simulink model "Pitch_Actuation_Hydraulic_Testrig_rt"  (Simulink 7.9)
settings: Solver=ode15s  StartTime=0.0  StopTime=10.0  RelTol=1e-3
PostLoadFcn:
  | warning off xPCTarget:sampleTime:sampleTimeInvariance;
  | warning off Simulink:SL_MdlFileShadowedByFile;
StartFcn:
  | tic;
StopFcn:
  | Elapsed_Sim_Time = toc; disp(['Elapsed time is ' num2str(Elapsed_Sim_Time)])
undefined symbols (not defined in the file or in its folder): sigbuilder_block, WT_Params
libraries: fl_lib x20, mblibv1 x12, nesl_utility x10, sh_lib x9, xpclib x1
Description:
  | Copyright 2011 The MathWorks, Inc.
settings Model: Creator=smiller  LastModifiedBy=smiller  ExtModeTrigDuration=200  BufferReuse=off
settings SolverCC: ExtrapolationOrder=2  NumberNewtonIterations=2  MaxConsecutiveMinStep=3
settings DataIOCC: LimitDataPoints=off
settings OptimizationCC: BlockReduction=off  OptimizeBlockIOStorage=off  BufferReuse=off  ExpressionFolding=off  LocalBlockOutputs=off
settings DebuggingCC: SolverPrmCheckMsg=none  FcnCallInpInsideContextMsg=Use local settings  UnconnectedInputMsg=none  UnconnectedOutputMsg=none  StrictBusMsg=Warning
settings HardwareCC: ProdIntDivRoundTo=Zero  ProdEndianess=LittleEndian  ProdHWDeviceType=Generic->32-bit x86 compatible
settings RTWCC: SystemTargetFile=xpctarget.tlc  TemplateMakefile=xpc_default_tmf  Description=xPC Target  ProcessScript=xpctarget_make_rtw_hook  RTWCompilerOptimization=On
settings xpcTargetCC: TargetFcnLib=ansi_tfl_table_tmw.mat  CodeReplacementLibrary=XPC_BLAS  CodeExecutionProfiling=off  ParMdlRefBuildCompliant=on  ConcurrentExecutionCompliant=on  CombineSignalStateStructs=off  PortableWordSizes=off  GRTInterface=on  xPCTaskExecutionProfile=off  xPCRL32EventNumber=5000  xPCLoadParamSetFile=off  xPCConcurrentTasks=off  xPCEnableSFAnimation=off
settings SimscapeCC: ExplicitSolverDiagnosticOptions=none
settings SimMechanicsCC: WarnOnRedundantConstraints=off  VisSampleTime=0.1  AnimationDelay=0  LastVizWinPosition=[420 528 560 420]  CamPosition=[-0.6;-13.224;-0.5;]  CamTarget=[-0.6;19.95;-0.5;]  CamUpVector=[0;0;1;]  CamHeight=3.468  VisBackgroundColor=[0.9;0.9;0.95;]  DefaultBodyColor=[1;0;0;]
settings ConfigurationSet: Description=SimMechanics 2G

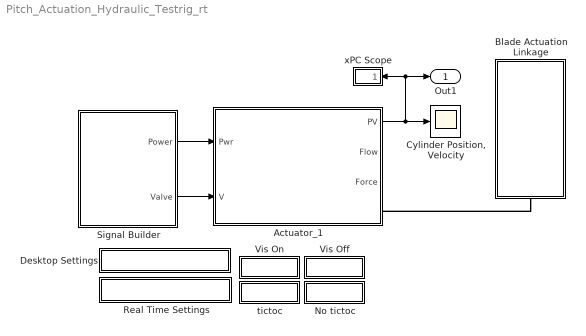
== system Pitch_Actuation_Hydraulic_Testrig_rt ==
  Actuator_1 : Subsystem
      mask Display: image(imread('Pitch_Hydraulic_Actuator_IMAGE.jpg'));
  Blade Actuation Linkage : Subsystem
      mask Display: image(imread('Single_Blade_IMAGE.jpg'));
  "Cylinder Position, Velocity" : Scope
      settings: TimeRange=10  YMin=-0.4  YMax=0.6  SaveName=Hydraulic_Testrig_DATA
  Desktop Settings : Subsystem
      settings: OpenFcn=|
      | set_param(bdroot,'Solver','ODE15s','MaxStep','auto');
      | 
      | tvar_solverBlock = find_system(bdroot, 'SubClassName', 'solver');
      | 
      | for i=1:size(tvar_solverBlock,1)
      | 
      | set_param(char(tvar_solverBlock(i)), 'UseLocalSolver','off','DoFixedCost','off');
      | end
      | 
      | clear tvar_solverBlock
      mask Display: disp('Desktop Settings')
  No tictoc : Subsystem
      settings: OpenFcn=|
      | set_param(bdroot,'StartFcn','');
      | set_param(bdroot,'StopFcn','');
      mask Display: disp('No tictoc')
  Real Time Settings : Subsystem
      settings: OpenFcn=|
      | tvar_Nonlinear_Iterations = '3';
      | 
      | tvar_StepSize = '0.005';
      | 
      | %tvar_LocalSolver = 'NE_TRAPEZOIDAL_ADVANCER';
      | 
      | tvar_LocalSolver = 'NE_BACKWARD_EULER_ADVANCER';
      | 
      | set_param(bdroot,'Solver','ode3','FixedStep','auto');
      | 
      | tvar_solverBlock = find_system(bdroot, 'SubClassName', 'solver');
      | for i=1:size(tvar_solverBlock,1)
      | 
      | set_param(char(tvar_solverBlock(i)), 'UseLocalSolver','on','DoFixedCost','on','MaxNonlinIter',tvar_Nonlinear_Iterations,'LocalSolverChoice',tvar_LocalSolver,'LocalSolverSampleTime',tvar_StepSize);
      | end
      | clear tvar_Nonlinear_Iterations tvar_StepSize tvar_LocalSolver tvar_solverBlock
      mask Display: disp('Real Time Settings')
  Signal Builder : Subsystem  Tag=STV Subsys  LoadFcn=sigbuilder_block('load');  StartFcn=sigbuilder_block('start');  StopFcn=sigbuilder_block('stop');  ClipboardFcn=sigbuilder_block('clipboard');  mask(Sigbuilder block){}
      mask help: Sigbuilder GUI
      mask init:
      | if ~strcmp(get_param(bdroot(gcbh),'SimulationStatus'),'stopped') tuvar = sigbuilder_block('maskInit'); end
      settings: CopyFcn=sigbuilder_block('copy');  DeleteFcn=sigbuilder_block('delete');  ModelCloseFcn=sigbuilder_block('modelClose');  PreSaveFcn=sigbuilder_block('preSave');  PauseFcn=sigbuilder_block('pause')  ContinueFcn=sigbuilder_block('continue')  NameChangeFcn=sigbuilder_block('namechange');  OpenFcn=sigbuilder_block('open',[141.75 274.5 550.5 399.75 ]);  CloseFcn=sigbuilder_block('close');
      mask Display: plot(0,0,100,100,[10,10,40,40,10],[80,20,20,80,80],[40,10],[50,50], [40,27,10],[65,72,56],[40,25,25,10],[28,28,43,43]);
  Vis Off : Subsystem
      settings: OpenFcn=|
      | Temp_ENVHa= get_param(find_system(gcs,'LookUnderMasks','all','FollowLinks','on','ClassName','Environment'),'handle');
      | 
      | set_param(Temp_ENVHa{1},'VisualizeMachine','off');
      | 
      | set_param(gcs,'VisDuringSimulation','off')
      | set_param(gcs,'VisOnUpdateDiagram','off')
      mask Display: disp('Vis Off')
  Vis On : Subsystem
      settings: OpenFcn=|
      | Temp_ENVHa= get_param(find_system(gcs,'LookUnderMasks','all','FollowLinks','on','ClassName','Environment'),'handle');
      | 
      | set_param(Temp_ENVHa{1},'VisualizeMachine','on');
      | clear Temp_ENVHa;
      | set_param(gcs,'VisDuringSimulation','on')
      | set_param(gcs,'VisOnUpdateDiagram','on')
      mask Display: disp('Vis On')
  tictoc : Subsystem
      settings: OpenFcn=|
      | set_param(bdroot,'StartFcn','tic;');
      | set_param(bdroot,'StopFcn','Elapsed_Sim_Time = toc; disp([''Elapsed time is '' num2str(Elapsed_Sim_Time)])');
      mask Display: disp('tictoc')
  xPC Scope : Subsystem
      mask Display: disp('xPC')
  Out1 : Outport
  wires:
  Signal Builder/1(Power) -> Actuator_1/1(Pwr)
  Signal Builder/2(Valve) -> Actuator_1/2(V)
  Actuator_1/1(PV) -> "Cylinder Position, Velocity"/1, Out1/1, xPC Scope/1(In1)
  connections:
  Blade Actuation Linkage/LConn1 -- Actuator_1/RConn1

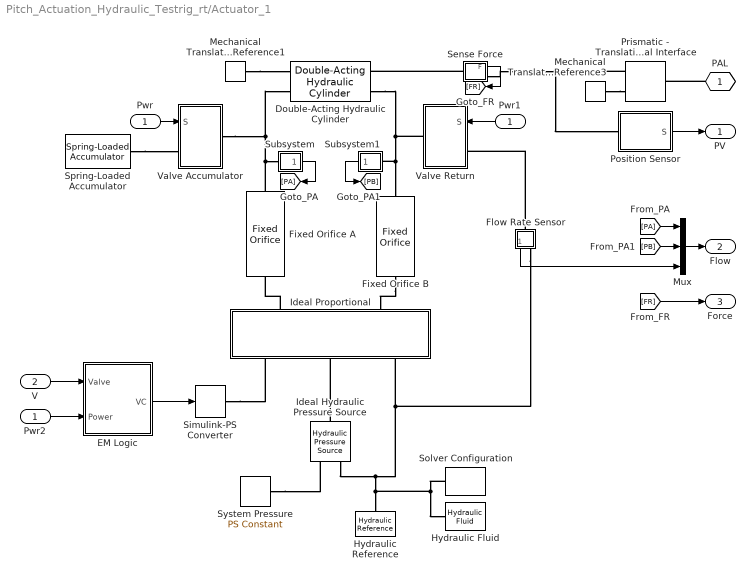
== system Pitch_Actuation_Hydraulic_Testrig_rt/Actuator_1 ==
  Pwr : Inport
  V : Inport  Port=2
  Double-Acting Hydraulic Cylinder : sh_lib/Hydraulic Cylinders/Double-Acting Hydraulic Cylinder  area_A=WT_Params.Pitch_Actuator.Cylinder.piston_area m^2  area_B=WT_Params.Pitch_Actuator.Cylinder.piston_area m^2  stroke=WT_Params.Pitch_Actuator.Cylinder.stroke m  init_pos=WT_Params.Pitch_Actuator.Cylinder.initial_disp_from_a m  dead_vol_A=1e-04 m^3  dead_vol_B=1e-04 m^3  init_pressure_A=0 Pa  init_pressure_B=0 Pa  k_sh=1.4  stiff=WT_Params.Pitch_Actuator.Cylinder.contact_stiffness N/m  D=WT_Params.Pitch_Actuator.Cylinder.contact_damping N/(m/s)  or=2  LocalVarLogging=[]
  EM Logic : Subsystem
  Fixed Orifice A : sh_lib/Orifices/Fixed Orifice  area=WT_Params.Pitch_Actuator.orifice_area m^2  C_d=0.7  Re_cr=12  flow_rate_Log=off  pr_drop_Log=off  Re_Log=off  power_Log=off  LocalVarNames=|flow_rate|pr_drop|Re|power  LocalVarDescs=|Flow rate through the orifice (m^3/s)|Pressure drop across the orifice (Pa)|Reynolds number|Power (W)  LocalVarLogging=[0 0 0 0]
  Fixed Orifice B : sh_lib/Orifices/Fixed Orifice  area=WT_Params.Pitch_Actuator.orifice_area m^2  C_d=0.7  Re_cr=12  flow_rate_Log=off  pr_drop_Log=off  Re_Log=off  power_Log=off  LocalVarNames=|flow_rate|pr_drop|Re|power  LocalVarDescs=|Flow rate through the orifice (m^3/s)|Pressure drop across the orifice (Pa)|Reynolds number|Power (W)  LocalVarLogging=[0 0 0 0]
  Flow Rate Sensor : Subsystem
      mask Display: disp('F')
  Hydraulic Reference : fl_lib/Hydraulic/Hydraulic Elements/Hydraulic Reference  q_Log=off  LocalVarNames=|q  LocalVarDescs=|q  LocalVarLogging=[]
  Hydraulic Fluid : sh_lib/Hydraulic Utilities/Hydraulic Fluid  DataSource=1  SelFluid=1  SysTemp=60 c  TrapAir=0.005  ViscDerFactor=1  LocalVarLogging=[]
  Ideal Proportional : Subsystem
      mask Display:
      | plot([198.418507352471;198.418507352471], [5.66910021007061;25.5109509453177])
      | plot([189.914857037365;206.922157667577], [25.5109509453177;25.5109509453177])
      | plot([240.936758928001;240.936758928001], [5.66910021007061;25.5109509453177])
      | plot([232.433108612895;249.440409243107], [25.5109509453177;25.5109509453177])
      | plot([240.936758928001;240.936758928001], [76.5328528359532;56.6910021007061])
      | plot([232.433108612895;249.440409243107], [56.6910021007061;56.6910021007061])
      | plot([198.418507352471;198.418507352471], [76.5328528359532;56.6910021007061])
      | plot([189.914857037365;206.922157667577], [56.6910021007061;56.6910021007061])
      | plot([99.2092536762357;99.2092536762357], [76.5328528359532;5.66910021007061])
      | plot([141.727505251765;141.727505251765], [76.5328528359532;5.66910021007061])
      | plot([170.073006302118;170.073006302118], [76.5328528359532;5.66910021007061])
      | plot([269.282259978354;269.282259978354], [76.5328528359532;5.66910021007061])
      | patch([99.2092536762357;93.5401534661651;104.878353886306;99.2092536762357], [76.5328528359532;53.8564519956708;53.8564519956708;76.5328528359532],[0 0 0])
      | plot([99.2092536762357;93.5401534661651;104.878353886306;99.2092536762357], [76.5328528359532;53.8564519956708;53.8564519956708;76.5328528359532])
      | patch([141.727505251765;136.058405041695;147.396605461836;141.727505251765], [5.66910021007061;28.3455010503531;28.3455010503531;5.66910021007061],[0 0 0])
      | plot([141.727505251765;136.058405041695;147.396605461836;141.727505251765], [5.66910021007061;28.3455010503531;28.3455010503531;5.66910021007061])
      | plot([297.627761028707;340.146012604237], [5.66910021007061;76.5328528359532])
      | plot([297.627761028707;340.146012604237], [76.5328528359532;5.66910021007061])
      | plot([70.8637526258826;368.49151365459;368.49151365459;70.8637526258826;70.8637526258826], [76.5328528359532;76.5328528359532;5.66910021007061;5.66910021007061;76.5328528359532])
      | patch([297.627761028707;303.296861238778;311.800511553884;297.627761028707], [5.66910021007061;25.5109509453177;19.8418507352471;5.66910021007061],[0 0 0])
      | plot([297.627761028707;303.296861238778;311.800511553884;297.627761028707], [5.66910021007061;25.5109509453177;19.8418507352471;5.66910021007061])
      | patch([297.627761028707;303.296861238778;311.800511553884;297.627761028707], [76.5328528359532;56.6910021007061;62.3601023107767;76.5328528359532],[0 0 0])
      | plot([297.627761028707;303.296861238778;311.800511553884;297.627761028707], [76.5328528359532;56.6910021007061;62.3601023107767;76.5328528359532])
      | plot([62.3601023107767;374.16061386466], [82.2019530460238;82.2019530460238])
      | plot([65.194652415812;376.995163969696], [0;0])
      | plot([70.8637526258826;0;0;70.8637526258826;70.8637526258826], [53.8564519956708;53.8564519956708;25.5109509453177;25.5109509453177;53.8564519956708]-25.5109509453177+5.66910021007061)
      | plot([70.8637526258826;0;0;70.8637526258826;70.8637526258826]+368.49151365459, [53.8564519956708;53.8564519956708;25.5109509453177;25.5109509453177;53.8564519956708]-25.5109509453177+5.66910021007061)
      | plot([15 25], [5.66910021007061 35])
      | plot([25 15]+405, [5.66910021007061 35])
      | plot([42.5 40]+5,[70 58]);
      | plot([45 50]+2.5,[70 45]);
      | plot([45 50]+7.5,[45 70]);
      | plot([45 50]+12.5,[70 45]);
      | plot([45 50]+17.5,[45 70]);
      | plot([40 42.5]+27.5,[70 58]);
      | plot([42.5 40]+5+324,[70 58]);
      | plot([45 50]+2.5+324,[70 45]);
      | plot([45 50]+7.5+324,[45 70]);
      | plot([45 50]+12.5+324,[70 45]);
      | plot([45 50]+17.5+324,[45 70]);
      | plot([40 42.5]+27.5+324,[70 58]);
      | ;color('red');
      | port_label('LConn', 1,'A')
      | port_label('LConn', 2,'B')
      | port_label('RConn', 1,'S')
      | port_label('RConn', 2,'P')
      | port_label('RConn', 3,'T')
  Ideal Hydraulic Pressure Source : fl_lib/Hydraulic/Hydraulic Sources/Hydraulic Pressure Source  q_Log=off  p_Log=off  LocalVarNames=|flow_rate|pr_differential|power  LocalVarDescs=|Flow rate through the source (m^3/s)|Pressure differential across the source (Pa)|Source power (W)  LocalVarLogging=[0 0 0]
  Mechanical Translational Reference1 : fl_lib/Mechanical/Translational Elements/Mechanical Translational Reference  Tag=Factory Generic  f_Log=off  LocalVarNames=|f  LocalVarDescs=|f  LocalVarLogging=[]
  Mechanical Translational Reference3 : fl_lib/Mechanical/Translational Elements/Mechanical Translational Reference  Tag=Factory Generic  f_Log=off  LocalVarNames=|f  LocalVarDescs=|f  LocalVarLogging=[]
  Mux : Mux  Inputs=3
  Position Sensor : Subsystem
      mask Display:
      | plot([25.5109509453177;56.6910021007061;70.8637526258826;96.3747035712004;127.554754726589;155.900255776942;184.245756827295;212.591257877648;235.26765871793;252.274959348142;283.455010503531], [155.900255776942;155.900255776942;110.547454096377;198.418507352471;113.382004201412;198.418507352471;116.216554306448;198.418507352471;113.382004201412;155.900255776942;155.900255776942])
      | plot([155.900255776942;155.900255776942], [266.447709873319;198.418507352471])
      | patch([155.900255776942;170.073006302118;141.727505251765;155.900255776942], [198.418507352471;226.764008402824;226.764008402824;198.418507352471], [0;0;0])
      | plot([155.900255776942;170.073006302118;141.727505251765;155.900255776942], [198.418507352471;226.764008402824;226.764008402824;198.418507352471])
      | ;
      | color('red');
      | port_label('LConn', 1,'R')
      | port_label('output', 1,'P')
  Prismatic - Translational Interface : mblibv1/Interface  Elements/Prismatic - Translational Interface  UpdateFromCAD=off  DialogClass=PrismaticTranslationalInterface  Primitive=P1
  Pwr1 : InportShadow  Port=1
  Pwr2 : InportShadow  Port=1
  Sense Force : Subsystem
      mask Display: disp('F');
  Simulink-PS Converter : nesl_utility/Simulink-PS Converter  PhysicalDomain=network_engine_domain  LeftPortType=input  RightPortType=output  SubClassName=ps_input  Unit=1  AffineConversion=off  InputFilterTimeConstant=.001  UdotUserProvided=0  SimscapeFilterOrder=1  InputFiltering=off
  Solver Configuration : nesl_utility/Solver Configuration  PhysicalDomain=network_engine_domain  LeftPortType=input  RightPortType=generic  SubClassName=solver  UseCustomDae=off  DoDC=off  ResidualTolerance=WT_Params.Pitch_Actuator.constraint_tol  UseLocalSolver=off  LocalSolverChoice=NE_BACKWARD_EULER_ADVANCER  LocalSolverSampleTime=0.005  DoFixedCost=off  MaxNonlinIter=3  MaxModeIter=2  LinearAlgebra=Full  Accelerate=off  Profile=off  UseLocalSampling=off  DelaysMemoryBudget=1024
  Spring-Loaded Accumulator : sh_lib/Accumulators/Spring-Loaded Accumulator  capacity=WT_Params.Pitch_Actuator.Accumulator.capacity m^3  pr_preload=WT_Params.Pitch_Actuator.Accumulator.preload_pressure Pa  pr_max=WT_Params.Pitch_Actuator.Accumulator.maximum_pressure Pa  v_init=WT_Params.Pitch_Actuator.Accumulator.initial_volume m^3  str_compl=4e-15 m^3/Pa  flow_rate_Log=off  pr_fluid_Log=off  fluid_volume_Log=off  LocalVarNames=|flow_rate|pr_fluid|fluid_volume  LocalVarDescs=|Accumulator flow rate (m^3/s)|Fluid pressure (Pa)|Initial fluid volume (m^3)  LocalVarLogging=[0 0 0]
  Subsystem : Subsystem
      mask Display: disp('P')
  Subsystem1 : Subsystem
      mask Display: disp('P')
  System Pressure : fl_lib/Physical Signals/Sources/PS Constant  constant=WT_Params.Pitch_Actuator.hydraulic_pressure  LocalVarLogging=[]
  Valve Accumulator : Subsystem
      mask Display:
      | plot([73.6983027309179;124.720204621553], [181.41120672226;181.41120672226])
      | plot([76.2808928266168;277.78591029346], [385.498814284801;385.498814284801])
      | plot([77.0997628569603;276.967040263116], [283.455010503531;283.455010503531])
      | plot([73.6983027309179;276.967040263116;276.967040263116;73.6983027309179;73.6983027309179], [487.542618066072;487.542618066072;79.3674029409885;79.3674029409885;487.542618066072])
      | plot([277.78591029346;226.764008402824], [181.41120672226;181.285226717591])
      | plot([226.764008402824;226.764008402824], [205.28441760689;157.286035828292])
      | patch([206.35524764657;206.35524764657;280.368500389159;206.35524764657], [400.805384851992;370.192243717611;385.498814284801;400.805384851992], [0;0;0])
      | plot([206.35524764657;206.35524764657;280.368500389159;206.35524764657], [400.805384851992;370.192243717611;385.498814284801;400.805384851992])
      | plot([124.720204621553;124.720204621553], [204.906477592885;156.971085816622])
      | plot([0;351.484213024378;351.484213024378;0;0], [566.910021007061;566.910021007061;0;0;566.910021007061])
      | ;
      | color('red');
      | port_label('input', 1,'S');
      | port_label('lconn', 1,'A');
      | port_label('rconn', 1,'B');
  Valve Return : Subsystem
      mask Display:
      | plot([73.6983027309179;124.720204621553], [181.41120672226;181.41120672226])
      | plot([76.2808928266168;277.78591029346], [385.498814284801;385.498814284801])
      | plot([77.0997628569603;276.967040263116], [283.455010503531;283.455010503531])
      | plot([73.6983027309179;276.967040263116;276.967040263116;73.6983027309179;73.6983027309179], [487.542618066072;487.542618066072;79.3674029409885;79.3674029409885;487.542618066072])
      | plot([277.78591029346;226.764008402824], [181.41120672226;181.285226717591])
      | plot([226.764008402824;226.764008402824], [205.28441760689;157.286035828292])
      | patch([206.35524764657;206.35524764657;280.368500389159;206.35524764657], [400.805384851992;370.192243717611;385.498814284801;400.805384851992], [0;0;0])
      | plot([206.35524764657;206.35524764657;280.368500389159;206.35524764657], [400.805384851992;370.192243717611;385.498814284801;400.805384851992])
      | plot([124.720204621553;124.720204621553], [204.906477592885;156.971085816622])
      | plot([0;351.484213024378;351.484213024378;0;0], [566.910021007061;566.910021007061;0;0;566.910021007061])
      | ;
      | color('red');
      | port_label('input', 1,'S');
      | port_label('lconn', 1,'A');
      | port_label('rconn', 1,'B');
  PAL : PMIOPort  Tag=PMCPort  Port=1  Side=Right
  PV : Outport
  Flow : Outport  Port=2
  Force : Outport  Port=3
  wires:
  [FR] -> Force/1
  Sense Force/1(F) -> [FR]
  Mux/1 -> Flow/1
  Position Sensor/1(S) -> PV/1
  Pwr/1 -> Valve Accumulator/1(S)
  Pwr1/1 -> Valve Return/1(S)
  V/1 -> EM Logic/1(Valve)
  Subsystem/1(P) -> [PA]
  Subsystem1/1(P) -> [PB]
  Flow Rate Sensor/1(Flow) -> Mux/3
  [PA] -> Mux/1
  [PB] -> Mux/2
  EM Logic/1(VC) -> Simulink-PS Converter/1
  Pwr2/1 -> EM Logic/2(Power)
  connections:
  Sense Force/LConn1 -- Double-Acting Hydraulic Cylinder/RConn1
  PAL/RConn1 -- Prismatic - Translational Interface/RConn1
  Mechanical Translational Reference3/LConn1 -- Prismatic - Translational Interface/LConn2
  System Pressure/RConn1 -- Ideal Hydraulic Pressure Source/RConn1
  Ideal Hydraulic Pressure Source/LConn1 -- Ideal Proportional/RConn2
  Simulink-PS Converter/RConn1 -- Ideal Proportional/RConn1
  Ideal Hydraulic Pressure Source/RConn2 -- Solver Configuration/RConn1 -- Hydraulic Fluid/RConn1 -- Hydraulic Reference/LConn1 -- Flow Rate Sensor/RConn1 -- Ideal Proportional/RConn3
  Fixed Orifice B/LConn1 -- Ideal Proportional/LConn2
  Ideal Proportional/LConn1 -- Fixed Orifice A/LConn1
  Double-Acting Hydraulic Cylinder/RConn2 -- Valve Return/RConn1 -- Fixed Orifice B/RConn1 -- Subsystem1/LConn1
  Fixed Orifice A/RConn1 -- Double-Acting Hydraulic Cylinder/LConn2 -- Valve Accumulator/RConn1 -- Subsystem/LConn1
  Mechanical Translational Reference1/LConn1 -- Double-Acting Hydraulic Cylinder/LConn1
  Spring-Loaded Accumulator/RConn1 -- Valve Accumulator/LConn1
  Sense Force/RConn1 -- Position Sensor/LConn1 -- Prismatic - Translational Interface/LConn1
  Flow Rate Sensor/LConn1 -- Valve Return/LConn1

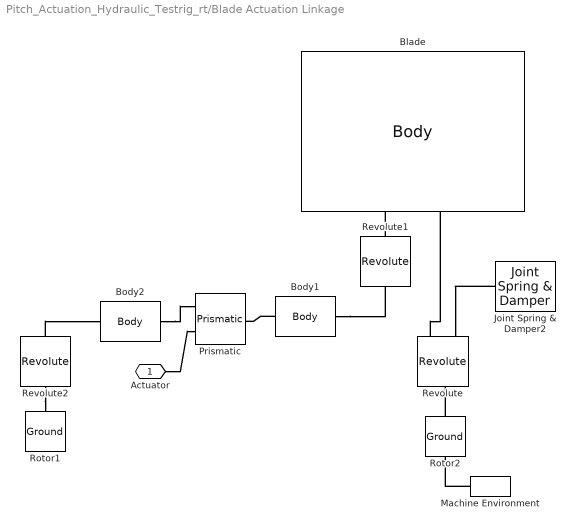
== system Pitch_Actuation_Hydraulic_Testrig_rt/Blade Actuation Linkage ==
  Blade : mblibv1/Bodies/Body  LConnTagsString=CS4|CS6|CS1|CS5  RConnTagsString=CS2  UpdateFromCAD=off  DialogClass=MechanicalBodyBlock  Mass=WT_Params.Blade.mass  MassUnits=kg  InertiaUnits=kg*m^2  Inertia=WT_Params.Blade.inertia  Shape=Cylinder  ShapeDims=[1 1]  ShapeUnits=m  ShapeUse=false  Density=1  DensityUnits=kg/m^3  DensityUse=false  GraphicsMode=MACHINE_DEFAULT  BodyColorSelMode=COLORPALETTE  BodyColor=[1 1 1]  AttachedToCS=CG  CG=Left$CG$[0 WT_Params.Blade.length/2 0]$CS1$CS1$m$[0 0 0]$Euler X-Y-Z$deg$CS1$false$none  WorkingFrames=Left$CS4$[0 0 0]$CS1$CS1$m$[0 0 0]$Euler X-Y-Z$deg$CS1$true$none#Left$CS6$[WT_Params.Blade.Actuator_Offset.x WT_Params.Blade.Actuator_Offset.y WT_Params.Blade.Actuator_Offset.z]$CS1$CS1$m$[0 0 0]$Euler X-Y-Z$deg$CS1$true$none#Left$CS1$[0 0 0]$Adjoining$Adjoining$m$[0 0 0]$Euler X-Y-Z$deg$Adjoining$true$none#Left$CS7$[WT_Params.Blade.Geometry.root_radius*sin(0) 0 WT_Params.Blade.Geometry.root_radius*cos(0)]$CS1$CS1$m$[0 0 0]$Euler X-Y-Z$deg$CS1$false$none#Left$CS8$[WT_Params.Blade.Geometry.root_radius*sin(0.2*pi) 0 WT_Params.Blade.Geometry.root_radius*cos(0.2*pi)]$CS1$CS1$m$[0 0 0]$Euler X-Y-Z$deg$CS1$false$none#Left$CS9$[WT_Params.Blade.Geometry.root_radius*sin(0.4*pi) 0 WT_Params.Blade.Geometry.root_radius*cos(0.4*pi)]$CS1$CS1$m$[0 0 0]$Euler X-Y-Z$deg$CS1$false$none#Left$CS10$[WT_Params.Blade.Geometry.root_radius*sin(0.6*pi) 0 WT_Params.Blade.Geometry.root_radius*cos(0.6*pi)]$CS1$CS1$m$[0 0 0]$Euler X-Y-Z$deg$CS1$false$none#Left$CS11$[WT_Params.Blade.Geometry.root_radius*sin(0.8*pi) 0 WT_Params.Blade.Geometry.root_radius*cos(0.8*pi)]$CS1$CS1$m$[0 0 0]$Euler X-Y-Z$deg$CS1$false$none#Left$CS12$[WT_Params.Blade.Geometry.root_radius*sin(1.0*pi) 0 WT_Params.Blade.Geometry.root_radius*cos(1.0*pi)]$CS1$CS1$m$[0 0 0]$Euler X-Y-Z$deg$CS1$false$none#Left$CS13$[WT_Params.Blade.Geometry.root_radius*sin(1.2*pi) 0 WT_Params.Blade.Geometry.root_radius*cos(1.2*pi)]$CS1$CS1$m$[0 0 0]$Euler X-Y-Z$deg$CS1$false$none#Left$CS14$[WT_Params.Blade.Geometry.root_radius*sin(1.4*pi) 0 WT_Params.Blade.Geometry.root_radius*cos(1.4*pi)]$CS1$CS1$m$[0 0 0]$Euler X-Y-Z$deg$CS1$false$none#Left$CS15$[WT_Params.Blade.Geometry.root_radius*sin(1.6*pi) 0 WT_Params.Blade.Geometry.root_radius*cos(1.6*pi)]$CS1$CS1$m$[0 0 0]$Euler X-Y-Z$deg$CS1$false$none#Left$CS16$[WT_Params.Blade.Geometry.root_radius*sin(1.8*pi) 0 WT_Params.Blade.Geometry.root_radius*cos(1.8*pi)]$CS1$CS1$m$[0 0 0]$Euler X-Y-Z$deg$CS1$false$none#Left$CS17$[0 WT_Params.Blade.length/4 0]$CS1$CS1$m$[0 0 0]$Euler X-Y-Z$deg$CS1$false$none#Left$CS18$[WT_Params.Blade.Geometry.ctr_to_leading_edge.x 0 WT_Params.Blade.Geometry.ctr_to_leading_edge.z]$CS17$CS17$m$[0 0 0]$Euler X-Y-Z$deg$CS1$false$none#Left$CS19$[WT_Params.Blade.Geometry.ctr_to_a1.x 0 WT_Params.Blade.Geometry.ctr_to_a1.z]$CS17$CS17$m$[0 0 0]$Euler X-Y-Z$deg$CS1$false$none#Left$CS20$[WT_Params.Blade.Geometry.ctr_to_a2.x 0 WT_Params.Blade.Geometry.ctr_to_a2.z]$CS17$CS17$m$[0 0 0]$Euler X-Y-Z$deg$CS1$false$none#Left$CS21$[WT_Params.Blade.Geometry.ctr_to_b1.x 0 WT_Params.Blade.Geometry.ctr_to_b1.z]$CS17$CS17$m$[0 0 0]$Euler X-Y-Z$deg$CS1$false$none#Left$CS25$[WT_Params.Blade.Geometry.ctr_to_b2.x 0 WT_Params.Blade.Geometry.ctr_to_b2.z]$CS17$CS17$m$[0 0 0]$Euler X-Y-Z$deg$CS1$false$none#Left$CS22$[WT_Params.Blade.Geometry.ctr_to_c1.x 0 WT_Params.Blade.Geometry.ctr_to_c1.z]$CS17$CS17$m$[0 0 0]$Euler X-Y-Z$deg$CS1$false$none#Left$CS3$[WT_Params.Blade.Geometry.ctr_to_d1.x 0 WT_Params.Blade.Geometry.ctr_to_d1.z]$CS17$CS17$m$[0 0 0]$Euler X-Y-Z$deg$CS1$false$none#Left$CS23$[WT_Params.Blade.Geometry.ctr_to_e1.x 0 WT_Params.Blade.Geometry.ctr_to_e1.z]$CS17$CS17$m$[0 0 0]$Euler X-Y-Z$deg$CS1$false$none#Left$CS24$[WT_Params.Blade.Geometry.ctr_to_trailing_edge.x 0 WT_Params.Blade.Geometry.ctr_to_trailing_edge.z]$CS17$CS17$m$[0 0 0]$Euler X-Y-Z$deg$CS1$false$none#Left$CS5$[0 0 0]$CS1$CS1$m$[0 0 0]$Euler X-Y-Z$deg$CS1$true$none#Right$CS2$[0 WT_Params.Blade.length 0]$CS1$CS1$m$[0 0 0]$Euler X-Y-Z$deg$CS1$true$none  CGPos=[0 WT_Params.Blade.length/2 0]  CGRot=[0 0 0]  CS0Pos=[]  CS0Rot=[]  CS1Pos=[0 0 0]  CS1Rot=[0 0 0]  CS2Pos=[0 WT_Params.Blade.length 0]  CS2Rot=[0 0 0]  CS3Pos=[WT_Params.Blade.Geometry.ctr_to_d1.x 0 WT_Params.Blade.Geometry.ctr_to_d1.z]  CS3Rot=[0 0 0]  CS4Pos=[0 0 0]  CS4Rot=[0 0 0]  CS5Pos=[0 0 0]  CS5Rot=[0 0 0]  CS6Pos=[WT_Params.Blade.Actuator_Offset.x WT_Params.Blade.Actuator_Offset.y WT_Params.Blade.Actuator_Offset.z]  CS6Rot=[0 0 0]  CS7Pos=[WT_Params.Blade.Geometry.root_radius*sin(0) 0 WT_Params.Blade.Geometry.root_radius*cos(0)]  CS7Rot=[0 0 0]  CS8Pos=[WT_Params.Blade.Geometry.root_radius*sin(0.2*pi) 0 WT_Params.Blade.Geometry.root_radius*cos(0.2*pi)]  CS8Rot=[0 0 0]  CS9Pos=[WT_Params.Blade.Geometry.root_radius*sin(0.4*pi) 0 WT_Params.Blade.Geometry.root_radius*cos(0.4*pi)]  CS9Rot=[0 0 0]  CS10Pos=[WT_Params.Blade.Geometry.root_radius*sin(0.6*pi) 0 WT_Params.Blade.Geometry.root_radius*cos(0.6*pi)]  CS10Rot=[0 0 0]  CS11Pos=[WT_Params.Blade.Geometry.root_radius*sin(0.8*pi) 0 WT_Params.Blade.Geometry.root_radius*cos(0.8*pi)]  CS11Rot=[0 0 0]  CS12Pos=[WT_Params.Blade.Geometry.root_radius*sin(1.0*pi) 0 WT_Params.Blade.Geometry.root_radius*cos(1.0*pi)]  CS12Rot=[0 0 0]  CS13Pos=[WT_Params.Blade.Geometry.root_radius*sin(1.2*pi) 0 WT_Params.Blade.Geometry.root_radius*cos(1.2*pi)]  CS13Rot=[0 0 0]  CS14Pos=[WT_Params.Blade.Geometry.root_radius*sin(1.4*pi) 0 WT_Params.Blade.Geometry.root_radius*cos(1.4*pi)]  CS14Rot=[0 0 0]  CS15Pos=[WT_Params.Blade.Geometry.root_radius*sin(1.6*pi) 0 WT_Params.Blade.Geometry.root_radius*cos(1.6*pi)]  CS15Rot=[0 0 0]  CS16Pos=[WT_Params.Blade.Geometry.root_radius*sin(1.8*pi) 0 WT_Params.Blade.Geometry.root_radius*cos(1.8*pi)]  CS16Rot=[0 0 0]  CS17Pos=[0 WT_Params.Blade.length/4 0]  CS17Rot=[0 0 0]  CS18Pos=[WT_Params.Blade.Geometry.ctr_to_leading_edge.x 0 WT_Params.Blade.Geometry.ctr_to_leading_edge.z]  CS18Rot=[0 0 0]  CS19Pos=[WT_Params.Blade.Geometry.ctr_to_a1.x 0 WT_Params.Blade.Geometry.ctr_to_a1.z]  CS19Rot=[0 0 0]  CS20Pos=[WT_Params.Blade.Geometry.ctr_to_a2.x 0 WT_Params.Blade.Geometry.ctr_to_a2.z]  CS20Rot=[0 0 0]
  Body1 : mblibv1/Bodies/Body  LConnTagsString=CS1  RConnTagsString=CS2  UpdateFromCAD=off  DialogClass=MechanicalBodyBlock  Mass=1  MassUnits=kg  InertiaUnits=kg*m^2  Inertia=eye(3)  Shape=Cylinder  ShapeDims=[1 1]  ShapeUnits=m  ShapeUse=false  Density=1  DensityUnits=kg/m^3  DensityUse=false  GraphicsMode=MACHINE_DEFAULT  BodyColorSelMode=MACHINE_DEFAULT  BodyColor=[1 0 0]  AttachedToCS=CG  CG=Left$CG$[-0.5 0 0]$CS1$CS1$m$[0 0 0]$Euler X-Y-Z$deg$WORLD$false$none  WorkingFrames=Left$CS1$[0 0 0]$Adjoining$Adjoining$m$[0 0 0]$Euler X-Y-Z$deg$WORLD$true$none#Right$CS2$[-1 0 0]$CS1$CS1$m$[0 0 0]$Euler X-Y-Z$deg$WORLD$true$none  CGPos=[-0.5 0 0]  CGRot=[0 0 0]  CS0Pos=[]  CS0Rot=[]  CS1Pos=[0 0 0]  CS1Rot=[0 0 0]  CS2Pos=[-1 0 0]  CS2Rot=[0 0 0]  CS3Pos=[]  CS3Rot=[]  CS4Pos=[]  CS4Rot=[]  CS5Pos=[]  CS5Rot=[]  CS6Pos=[]  CS6Rot=[]  CS7Pos=[]  CS7Rot=[]  CS8Pos=[]  CS8Rot=[]  CS9Pos=[]  CS9Rot=[]  CS10Pos=[]  CS10Rot=[]  CS11Pos=[]  CS11Rot=[]  CS12Pos=[]  CS12Rot=[]  CS13Pos=[]  CS13Rot=[]  CS14Pos=[]  CS14Rot=[]  CS15Pos=[]  CS15Rot=[]  CS16Pos=[]  CS16Rot=[]  CS17Pos=[]  CS17Rot=[]  CS18Pos=[]  CS18Rot=[]  CS19Pos=[]  CS19Rot=[]  CS20Pos=[]  CS20Rot=[]
  Body2 : mblibv1/Bodies/Body  LConnTagsString=CS1  RConnTagsString=CS2  UpdateFromCAD=off  DialogClass=MechanicalBodyBlock  Mass=1  MassUnits=kg  InertiaUnits=kg*m^2  Inertia=eye(3)  Shape=Cylinder  ShapeDims=[1 1]  ShapeUnits=m  ShapeUse=false  Density=1  DensityUnits=kg/m^3  DensityUse=false  GraphicsMode=MACHINE_DEFAULT  BodyColorSelMode=MACHINE_DEFAULT  BodyColor=[1 0 0]  AttachedToCS=CG  CG=Left$CG$[-0.5 0 0]$CS1$CS1$m$[0 0 0]$Euler X-Y-Z$deg$WORLD$false$none  WorkingFrames=Left$CS1$[0 0 0]$Adjoining$Adjoining$m$[0 0 0]$Euler X-Y-Z$deg$WORLD$true$none#Right$CS2$[-1 0 0]$CS1$CS1$m$[0 0 0]$Euler X-Y-Z$deg$WORLD$true$none  CGPos=[-0.5 0 0]  CGRot=[0 0 0]  CS0Pos=[]  CS0Rot=[]  CS1Pos=[0 0 0]  CS1Rot=[0 0 0]  CS2Pos=[-1 0 0]  CS2Rot=[0 0 0]  CS3Pos=[]  CS3Rot=[]  CS4Pos=[]  CS4Rot=[]  CS5Pos=[]  CS5Rot=[]  CS6Pos=[]  CS6Rot=[]  CS7Pos=[]  CS7Rot=[]  CS8Pos=[]  CS8Rot=[]  CS9Pos=[]  CS9Rot=[]  CS10Pos=[]  CS10Rot=[]  CS11Pos=[]  CS11Rot=[]  CS12Pos=[]  CS12Rot=[]  CS13Pos=[]  CS13Rot=[]  CS14Pos=[]  CS14Rot=[]  CS15Pos=[]  CS15Rot=[]  CS16Pos=[]  CS16Rot=[]  CS17Pos=[]  CS17Rot=[]  CS18Pos=[]  CS18Rot=[]  CS19Pos=[]  CS19Rot=[]  CS20Pos=[]  CS20Rot=[]
  Joint Spring & Damper2 : mblibv1/Force  Elements/Joint Spring & Damper  UpdateFromCAD=off  DialogClass=JointSpringDamper  JFEParameters=P1$false$0$0$0$m$m/s$N$deg$deg/s$N*m#P2$false$0$0$0$m$m/s$N$deg$deg/s$N*m#P3$false$0$0$0$m$m/s$N$deg$deg/s$N*m#R1$true$0$WT_Params.Blade.damping$0$m$m/s$N$deg$deg/s$N*m#R2$false$0$0$0$m$m/s$N$deg$deg/s$N*m#R3$false$0$0$0$m$m/s$N$deg$deg/s$N*m#S$false$0$0$0$m$m/s$N$deg$deg/s$N*m
  Machine Environment : mblibv1/Bodies/Machine Environment  PortType=env  PhysicalDomain=Mechanical  DialogTemplateClass=MECH.MachineEnvironment  SyncWhenCopied=off  Gravity=[0 -9.81 0]  GravityUnits=m/s^2  GravityAsSignal=off  Dimensionality=Auto-detect  AnalysisType=Forward dynamics  LinearAssemblyTolerance=1e-3  LinearAssemblyToleranceUnits=m  AngularAssemblyTolerance=1e-3  AngularAssemblyToleranceUnits=rad  ConstraintSolverType=Stabilizing  ConstraintRelTolerance=1e-4  ConstraintAbsTolerance=1e-4  UseRobustSingularityHandling=off  RedundancyAnalysisToleranceType=Automatically select tolerance  RedundancyAnalysisTolerance=1e-14  StatePerturbationType=Fixed  PerturbationSize=1e-5  VisualizeMachine=off  BodyVisualizationType=Use model default body geometries  BodyColorSelMode=Use model default  DefaultBodyColor=[1 0 0]
  Prismatic : mblibv1/Joints/Prismatic  LConnTagsString=__newl0|SA1  RConnTagsString=__newr0  UpdateFromCAD=off  NumSAPorts=1  CutJoint=off  MarkAsCut=off  Primitives=prismatic  PrimitiveProps=P1$World$[1 0 0]$prismatic  DialogClass=JointBlock  P1Axis=[1 0 0]
  Revolute : mblibv1/Joints/Revolute  LConnTagsString=__newl0|SA1  RConnTagsString=__newr0  UpdateFromCAD=off  NumSAPorts=1  CutJoint=off  MarkAsCut=off  Primitives=prismatic  PrimitiveProps=R1$World$[0 1 0]$revolute  DialogClass=JointBlock  R1Axis=[0 1 0]
  Revolute1 : mblibv1/Joints/Revolute  LConnTagsString=__newl0  RConnTagsString=__newr0  UpdateFromCAD=off  NumSAPorts=0  CutJoint=off  MarkAsCut=off  Primitives=prismatic  PrimitiveProps=R1$World$[0 1 0]$revolute  DialogClass=JointBlock  R1Axis=[0 1 0]
  Revolute2 : mblibv1/Joints/Revolute  LConnTagsString=__newl0  RConnTagsString=__newr0  UpdateFromCAD=off  NumSAPorts=0  CutJoint=off  MarkAsCut=off  Primitives=prismatic  PrimitiveProps=R1$World$[0 1 0]$revolute  DialogClass=JointBlock  R1Axis=[0 1 0]
  Rotor1 : mblibv1/Bodies/Ground  UpdateFromCAD=off  LeftPortType=env  RightPortType=workingframe  PhysicalDomain=Mechanical  DialogClass=GroundBlock  CoordPosition=[-2 -0.1 0.5]  CoordPositionUnits=m  StateVectorMgrId=-1  MachineId=[0 0]  ShowEnvPort=off
  Rotor2 : mblibv1/Bodies/Ground  UpdateFromCAD=off  LeftPortType=env  RightPortType=workingframe  PhysicalDomain=Mechanical  DialogClass=GroundBlock  CoordPosition=[0 0 0]  CoordPositionUnits=m  StateVectorMgrId=-1  MachineId=[0 0]  ShowEnvPort=on
  Actuator : PMIOPort  Port=1  Side=Left
  connections:
  Revolute1/LConn1 -- Blade/LConn2
  Revolute/LConn1 -- Blade/LConn3
  Body1/LConn1 -- Revolute1/RConn1
  Body1/RConn1 -- Prismatic/RConn1
  Body2/LConn1 -- Prismatic/LConn1
  Revolute2/LConn1 -- Body2/RConn1
  Machine Environment/RConn1 -- Rotor2/LConn1
  Rotor2/RConn1 -- Revolute/RConn1
  Revolute2/RConn1 -- Rotor1/RConn1
  Actuator/RConn1 -- Prismatic/LConn2
  Joint Spring & Damper2/LConn1 -- Revolute/LConn2

== system Pitch_Actuation_Hydraulic_Testrig_rt/Desktop Settings ==

== system Pitch_Actuation_Hydraulic_Testrig_rt/No tictoc ==

== system Pitch_Actuation_Hydraulic_Testrig_rt/Real Time Settings ==

== system Pitch_Actuation_Hydraulic_Testrig_rt/Signal Builder ==
  Demux : Demux  Tag=STV Demux  Outputs=2
  FromWs : FromWorkspace  Tag=STV FromWs  VariableName=tuvar  SampleTime=0  SigBuilderData=DataTag2  VnvData=DataTag3
      SigBuilderData=|
      | common.afterFinalStr = 'Extrapolate'
      | common.sampleTime = 0
      | dataSet.timeRange = [0 10]
      | dataSet.name = 'Group 1'
      | sbobj.Groups.Name = 'Group 1'
      | sbobj.Groups.Signals(1).Name = 'Power'
      | sbobj.Groups.Signals(1).XData = [0 4 6 6 10]
      | sbobj.Groups.Signals(1).YData = [24 24 24 0 0]
      | sbobj.Groups.Signals(2).Name = 'Valve'
      | sbobj.Groups.Signals(2).XData = [0 1 1 1.5 1.5 3 3 3.5 3.5 10]
      | sbobj.Groups.Signals(2).YData = [0 0 -1e-05 -1e-05 0 0 1e-05 1e-05 0 0]
  Power : Outport  Tag=STV Outport
  Valve : Outport  Tag=STV Outport  Port=2
  wires:
  Demux/1 -> Power/1
  FromWs/1 -> Demux/1
  Demux/2 -> Valve/1

== system Pitch_Actuation_Hydraulic_Testrig_rt/Vis Off ==

== system Pitch_Actuation_Hydraulic_Testrig_rt/Vis On ==

== system Pitch_Actuation_Hydraulic_Testrig_rt/tictoc ==

== system Pitch_Actuation_Hydraulic_Testrig_rt/xPC Scope ==
  In1 : Inport
  "Scope (xPC) " : xpclib/Misc./Scope (xPC)   scopeno=1  scopetype=Target  autostart=on  viewmode=Graphical redraw  formatstr='%15.6f'  grid=on  ylimits=[-0.4,0.6]  nosamples=200  noprepostsamples=0  interleave=1  triggermode=FreeRun  triggersignal=1  triggerlevel=0.0  triggerslope=Either  triggerscope=1  triggersample=0  filename=data.dat  mode=Lazy  writesize=512  autorestart=off  dynamicfilemode=off  maxwritefilesize=512*1024^2
  wires:
  In1/1 -> "Scope (xPC) "/1

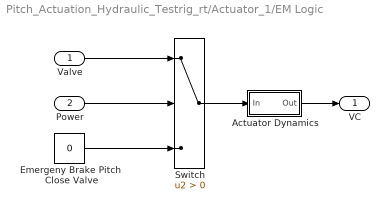
== system Pitch_Actuation_Hydraulic_Testrig_rt/Actuator_1/EM Logic ==
  Valve : Inport
  Power : Inport  Port=2
  Actuator Dynamics : Subsystem  mask(First-order lag supporting vector signals){b=WT_Params.Pitch_Actuator.hydraulic_actuator_time_constant, x_initial=0}
      mask prompts: b "Filter time constant"; x_initial "Initial output"
      mask help: Models a lag of the form 1/(b*s+1) where s is the Laplace operator.
  Emergeny Brake Pitch  Close Valve : Constant  Value=0
  Switch : Switch  Criteria=u2 > Threshold
  VC : Outport
  wires:
  Actuator Dynamics/1(Out) -> VC/1
  Valve/1 -> Switch/1
  Power/1 -> Switch/2
  Emergeny Brake Pitch  Close Valve/1 -> Switch/3
  Switch/1 -> Actuator Dynamics/1(In)

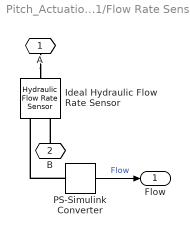
== system Pitch_Actuation_Hydraulic_Testrig_rt/Actuator_1/Flow Rate Sensor ==
  Ideal Hydraulic Flow Rate Sensor : fl_lib/Hydraulic/Hydraulic Sensors/Hydraulic Flow Rate Sensor  q_Log=off  p_Log=off  LocalVarNames=|q|p  LocalVarDescs=|q|p  LocalVarLogging=[]
  PS-Simulink Converter : nesl_utility/PS-Simulink Converter  PhysicalDomain=network_engine_domain  LeftPortType=input  RightPortType=output  SubClassName=ps_output  Unit=1  AffineConversion=off
  A : PMIOPort  Port=1  Side=Left
  B : PMIOPort  Port=2  Side=Right
  Flow : Outport
  wires:
  PS-Simulink Converter/1 -> Flow/1  "Flow"
  connections:
  PS-Simulink Converter/LConn1 -- Ideal Hydraulic Flow Rate Sensor/RConn1
  A/RConn1 -- Ideal Hydraulic Flow Rate Sensor/LConn1
  B/RConn1 -- Ideal Hydraulic Flow Rate Sensor/RConn2

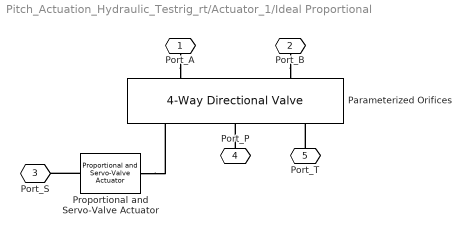
== system Pitch_Actuation_Hydraulic_Testrig_rt/Actuator_1/Ideal Proportional ==
  Parameterized Orifices : sh_lib/Valves/Directional Valves/4-Way Directional Valve  mdl_type=1  area_max=WT_Params.Pitch_Actuator.Valve.max_area m^2  opening_max=WT_Params.Pitch_Actuator.Valve.max_opening m  opening_tab="[  -0.002 0 0.002 0.005 0.015 ] m"  area_tab="[  1e-09 2.0352e-07 4.0736e-05 0.00011438 0.00034356 ] m^2"  pressure_tab="[  -1e+07 -5e+06 -2e+06 2e+06 5e+06 1e+07 ] Pa"  flow_rate_tab="[  -1e-07 -7.0711e-08 -4.4721e-08 4.4721e-08 7.0711e-08 1e-07 ; -2.0352e-05 -1.4391e-05 -9.1017e-06 9.1017e-06 1.4391e-05 2.0352e-05 ; -0.0040736 -0.0028805 -0.0018218 0.0018218 0.0028805 0.0040736 ; -0.011438 -0.0080879 -0.0051152 0.0051152 0.0080879 0.011438 ; -0.034356 -0.024293 -0.015364 0.015364 0.024293 0.034356 ; ] m^3/s"  interp_method=1  extrap_method=1  C_d=0.7  x_0_P_A=WT_Params.Pitch_Actuator.Valve.initial_opening_pa m  x_0_P_B=WT_Params.Pitch_Actuator.Valve.initial_opening_pb m  x_0_A_T=WT_Params.Pitch_Actuator.Valve.initial_opening_at m  x_0_B_T=WT_Params.Pitch_Actuator.Valve.initial_opening_bt m  Re_cr=12  A_leak=WT_Params.Pitch_Actuator.Valve.leakage_area m^2  LocalVarLogging=[]
  Proportional and Servo-Valve Actuator : sh_lib/Valves/Valve Actuators/Proportional and Servo-Valve Actuator  gain=WT_Params.Pitch_Actuator.Servo.gain  time_constant=WT_Params.Pitch_Actuator.Servo.time_constant s  saturation=WT_Params.Pitch_Actuator.Servo.saturation  LocalVarLogging=[]
  Port_A : PMIOPort  Port=1  Side=Left
  Port_B : PMIOPort  Port=2  Side=Left
  Port_S : PMIOPort  Port=3  Side=Right
  Port_P : PMIOPort  Port=4  Side=Right
  Port_T : PMIOPort  Port=5  Side=Right
  connections:
  Proportional and Servo-Valve Actuator/LConn1 -- Port_S/RConn1
  Port_T/RConn1 -- Parameterized Orifices/RConn3
  Port_P/RConn1 -- Parameterized Orifices/RConn2
  Proportional and Servo-Valve Actuator/RConn1 -- Parameterized Orifices/RConn1
  Port_B/RConn1 -- Parameterized Orifices/LConn2
  Port_A/RConn1 -- Parameterized Orifices/LConn1

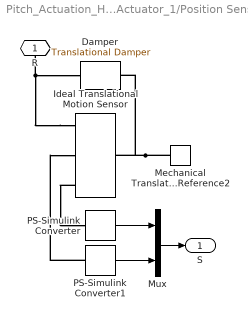
== system Pitch_Actuation_Hydraulic_Testrig_rt/Actuator_1/Position Sensor ==
  Damper : fl_lib/Mechanical/Translational Elements/Translational Damper  D=WT_Params.Pitch_Actuator.Cylinder.damping N/(m/s)  f_Log=off  v_Log=off  LocalVarNames=|force|rel_velocity|power  LocalVarDescs=|Damping force (N)|Damper relative velocity (m/s)|Power dissipated in the damper (W)  LocalVarLogging=[0 0 0]
  Ideal Translational Motion Sensor : fl_lib/Mechanical/Mechanical Sensors/Ideal Translational Motion Sensor  offset=WT_Params.Pitch_Actuator.Sensor.initial_position m  v_Log=off  f_Log=off  x_Log=off  LocalVarNames=|v|f|x  LocalVarDescs=|v|f|x  LocalVarLogging=[]
  Mechanical Translational Reference2 : fl_lib/Mechanical/Translational Elements/Mechanical Translational Reference  Tag=Factory Generic  f_Log=off  LocalVarNames=|f  LocalVarDescs=|f  LocalVarLogging=[]
  Mux : Mux  Inputs=2
  PS-Simulink Converter : nesl_utility/PS-Simulink Converter  PhysicalDomain=network_engine_domain  LeftPortType=input  RightPortType=output  SubClassName=ps_output  Unit=1  AffineConversion=off
  PS-Simulink Converter1 : nesl_utility/PS-Simulink Converter  PhysicalDomain=network_engine_domain  LeftPortType=input  RightPortType=output  SubClassName=ps_output  Unit=1  AffineConversion=off
  R : PMIOPort  Port=1  Side=Left
  S : Outport
  wires:
  PS-Simulink Converter/1 -> Mux/1
  Mux/1 -> S/1
  PS-Simulink Converter1/1 -> Mux/2
  connections:
  Ideal Translational Motion Sensor/RConn1 -- Damper/LConn1 -- R/RConn1
  Ideal Translational Motion Sensor/LConn1 -- Damper/RConn1 -- Mechanical Translational Reference2/LConn1
  Ideal Translational Motion Sensor/RConn3 -- PS-Simulink Converter/LConn1
  PS-Simulink Converter1/LConn1 -- Ideal Translational Motion Sensor/RConn2

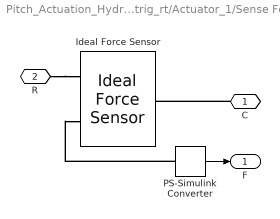
== system Pitch_Actuation_Hydraulic_Testrig_rt/Actuator_1/Sense Force ==
  Ideal Force Sensor : fl_lib/Mechanical/Mechanical Sensors/Ideal Force Sensor  v_Log=off  f_Log=off  LocalVarNames=|v|f  LocalVarDescs=|v|f  LocalVarLogging=[]
  PS-Simulink Converter : nesl_utility/PS-Simulink Converter  PhysicalDomain=network_engine_domain  LeftPortType=input  RightPortType=output  SubClassName=ps_output  Unit=1  AffineConversion=off
  C : PMIOPort  Port=1  Side=Right
  R : PMIOPort  Port=2  Side=Left
  F : Outport
  wires:
  PS-Simulink Converter/1 -> F/1
  connections:
  R/RConn1 -- Ideal Force Sensor/RConn1
  C/RConn1 -- Ideal Force Sensor/LConn1
  PS-Simulink Converter/LConn1 -- Ideal Force Sensor/RConn2

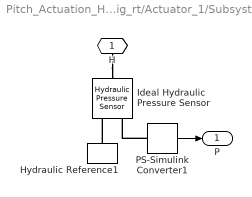
== system Pitch_Actuation_Hydraulic_Testrig_rt/Actuator_1/Subsystem ==
  Hydraulic Reference1 : fl_lib/Hydraulic/Hydraulic Elements/Hydraulic Reference  q_Log=off  LocalVarNames=|q  LocalVarDescs=|q  LocalVarLogging=[]
  Ideal Hydraulic Pressure Sensor : fl_lib/Hydraulic/Hydraulic Sensors/Hydraulic Pressure Sensor  q_Log=off  p_Log=off  LocalVarNames=|q|p  LocalVarDescs=|q|p  LocalVarLogging=[]
  PS-Simulink Converter1 : nesl_utility/PS-Simulink Converter  PhysicalDomain=network_engine_domain  LeftPortType=input  RightPortType=output  SubClassName=ps_output  Unit=1  AffineConversion=off
  H : PMIOPort  Port=1  Side=Left
  P : Outport
  wires:
  PS-Simulink Converter1/1 -> P/1
  connections:
  Hydraulic Reference1/LConn1 -- Ideal Hydraulic Pressure Sensor/RConn1
  PS-Simulink Converter1/LConn1 -- Ideal Hydraulic Pressure Sensor/RConn2
  H/RConn1 -- Ideal Hydraulic Pressure Sensor/LConn1

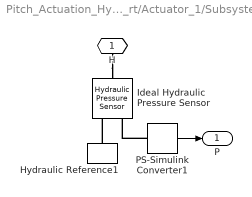
== system Pitch_Actuation_Hydraulic_Testrig_rt/Actuator_1/Subsystem1 ==
  Hydraulic Reference1 : fl_lib/Hydraulic/Hydraulic Elements/Hydraulic Reference  q_Log=off  LocalVarNames=|q  LocalVarDescs=|q  LocalVarLogging=[]
  Ideal Hydraulic Pressure Sensor : fl_lib/Hydraulic/Hydraulic Sensors/Hydraulic Pressure Sensor  q_Log=off  p_Log=off  LocalVarNames=|q|p  LocalVarDescs=|q|p  LocalVarLogging=[]
  PS-Simulink Converter1 : nesl_utility/PS-Simulink Converter  PhysicalDomain=network_engine_domain  LeftPortType=input  RightPortType=output  SubClassName=ps_output  Unit=1  AffineConversion=off
  H : PMIOPort  Port=1  Side=Left
  P : Outport
  wires:
  PS-Simulink Converter1/1 -> P/1
  connections:
  H/RConn1 -- Ideal Hydraulic Pressure Sensor/LConn1
  PS-Simulink Converter1/LConn1 -- Ideal Hydraulic Pressure Sensor/RConn2
  Hydraulic Reference1/LConn1 -- Ideal Hydraulic Pressure Sensor/RConn1

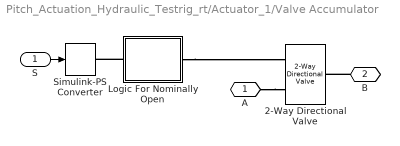
== system Pitch_Actuation_Hydraulic_Testrig_rt/Actuator_1/Valve Accumulator ==
  S : Inport
  2-Way Directional Valve : sh_lib/Valves/Directional Valves/2-Way Directional Valve  mdl_type=1  area_max=WT_Params.Pitch_Actuator.Emergency_Pitch_Valve.max_area m^2  opening_max=0.005 m  opening_tab="[  -0.002 0 0.002 0.005 0.015 ] m"  area_tab="[  1e-09 2.0352e-07 4.0736e-05 0.00011438 0.00034356 ] m^2"  pressure_tab="[  -1e+07 -5e+06 -2e+06 2e+06 5e+06 1e+07 ] Pa"  flow_rate_tab="[  -1e-07 -7.0711e-08 -4.4721e-08 4.4721e-08 7.0711e-08 1e-07 ; -2.0352e-05 -1.4391e-05 -9.1017e-06 9.1017e-06 1.4391e-05 2.0352e-05 ; -0.0040736 -0.0028805 -0.0018218 0.0018218 0.0028805 0.0040736 ; -0.011438 -0.0080879 -0.0051152 0.0051152 0.0080879 0.011438 ; -0.034356 -0.024293 -0.015364 0.015364 0.024293 0.034356 ; ] m^3/s"  interp_method=1  extrap_method=1  C_d=0.7  x_0=0 m  Re_cr=12  A_leak=1e-12 m^2  LocalVarLogging=[]
  Logic For Nominally Open : Subsystem
  Simulink-PS Converter : nesl_utility/Simulink-PS Converter  PhysicalDomain=network_engine_domain  LeftPortType=input  RightPortType=output  SubClassName=ps_input  Unit=1  AffineConversion=off  InputFilterTimeConstant=.001  UdotUserProvided=0  SimscapeFilterOrder=1  InputFiltering=off
  A : PMIOPort  Port=1  Side=Left
  B : PMIOPort  Port=2  Side=Right
  wires:
  S/1 -> Simulink-PS Converter/1
  connections:
  Logic For Nominally Open/LConn1 -- Simulink-PS Converter/RConn1
  A/RConn1 -- 2-Way Directional Valve/LConn2
  B/RConn1 -- 2-Way Directional Valve/RConn1
  Logic For Nominally Open/RConn1 -- 2-Way Directional Valve/LConn1

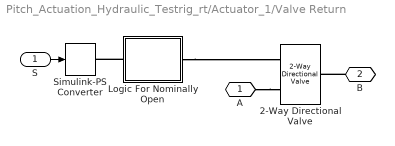
== system Pitch_Actuation_Hydraulic_Testrig_rt/Actuator_1/Valve Return ==
  S : Inport
  2-Way Directional Valve : sh_lib/Valves/Directional Valves/2-Way Directional Valve  mdl_type=1  area_max=WT_Params.Pitch_Actuator.Emergency_Pitch_Valve.max_area m^2  opening_max=0.005 m  opening_tab="[  -0.002 0 0.002 0.005 0.015 ] m"  area_tab="[  1e-09 2.0352e-07 4.0736e-05 0.00011438 0.00034356 ] m^2"  pressure_tab="[  -1e+07 -5e+06 -2e+06 2e+06 5e+06 1e+07 ] Pa"  flow_rate_tab="[  -1e-07 -7.0711e-08 -4.4721e-08 4.4721e-08 7.0711e-08 1e-07 ; -2.0352e-05 -1.4391e-05 -9.1017e-06 9.1017e-06 1.4391e-05 2.0352e-05 ; -0.0040736 -0.0028805 -0.0018218 0.0018218 0.0028805 0.0040736 ; -0.011438 -0.0080879 -0.0051152 0.0051152 0.0080879 0.011438 ; -0.034356 -0.024293 -0.015364 0.015364 0.024293 0.034356 ; ] m^3/s"  interp_method=1  extrap_method=1  C_d=0.7  x_0=0 m  Re_cr=12  A_leak=1e-12 m^2  LocalVarLogging=[]
  Logic For Nominally Open : Subsystem
  Simulink-PS Converter : nesl_utility/Simulink-PS Converter  PhysicalDomain=network_engine_domain  LeftPortType=input  RightPortType=output  SubClassName=ps_input  Unit=1  AffineConversion=off  InputFilterTimeConstant=.001  UdotUserProvided=0  SimscapeFilterOrder=1  InputFiltering=off
  A : PMIOPort  Port=1  Side=Left
  B : PMIOPort  Port=2  Side=Right
  wires:
  S/1 -> Simulink-PS Converter/1
  connections:
  Logic For Nominally Open/RConn1 -- 2-Way Directional Valve/LConn1
  B/RConn1 -- 2-Way Directional Valve/RConn1
  A/RConn1 -- 2-Way Directional Valve/LConn2
  Logic For Nominally Open/LConn1 -- Simulink-PS Converter/RConn1

== system Pitch_Actuation_Hydraulic_Testrig_rt/Actuator_1/EM Logic/Actuator Dynamics ==
  In : Inport
  Gain : Gain  Gain=1/b
  Integrator : Integrator  InitialCondition=x_initial
  Sum : Sum  Inputs=|+-  SaturateOnIntegerOverflow=on  InputSameDT=on  OutDataTypeStr=Inherit: Same as first input
  Out : Outport
  wires:
  Sum/1 -> Integrator/1
  In/1 -> Sum/1
  Integrator/1 -> Gain/1
  Gain/1 -> Sum/2, Out/1

== system Pitch_Actuation_Hydraulic_Testrig_rt/Actuator_1/Valve Accumulator/Logic For Nominally Open ==
  PS Gain : fl_lib/Physical Signals/Functions/PS Gain  gain=-1  LocalVarLogging=[]
  PS Subtract : fl_lib/Physical Signals/Functions/PS Subtract  LocalVarLogging=[]
  Voltage_Open : fl_lib/Physical Signals/Sources/PS Constant  constant=24  LocalVarLogging=[]
  S : PMIOPort  Port=1  Side=Left
  VA : PMIOPort  Port=2  Side=Right
  connections:
  PS Subtract/LConn2 -- Voltage_Open/RConn1
  PS Subtract/RConn1 -- PS Gain/LConn1
  S/RConn1 -- PS Subtract/LConn1
  VA/RConn1 -- PS Gain/RConn1

== system Pitch_Actuation_Hydraulic_Testrig_rt/Actuator_1/Valve Return/Logic For Nominally Open ==
  PS Gain : fl_lib/Physical Signals/Functions/PS Gain  gain=-1  LocalVarLogging=[]
  PS Subtract : fl_lib/Physical Signals/Functions/PS Subtract  LocalVarLogging=[]
  Voltage_Open : fl_lib/Physical Signals/Sources/PS Constant  constant=24  LocalVarLogging=[]
  S : PMIOPort  Port=1  Side=Left
  VA : PMIOPort  Port=2  Side=Right
  connections:
  VA/RConn1 -- PS Gain/RConn1
  S/RConn1 -- PS Subtract/LConn1
  PS Subtract/RConn1 -- PS Gain/LConn1
  PS Subtract/LConn2 -- Voltage_Open/RConn1
